simulink model "invDyn"  (R2021a)
settings: Solver=VariableStepAuto  StartTime=0.0  StopTime=60  RelTol=1e-3
values from neighbouring files (symbols this model uses):
  kd = eye(3)*40    [params.m]
  kp = eye(3)*1000    [params.m]
settings Model: Creator=antoninoparisi  LastModifiedBy=antoninoparisi
settings DebuggingCC: UnderSpecifiedDimensionMsg=warning

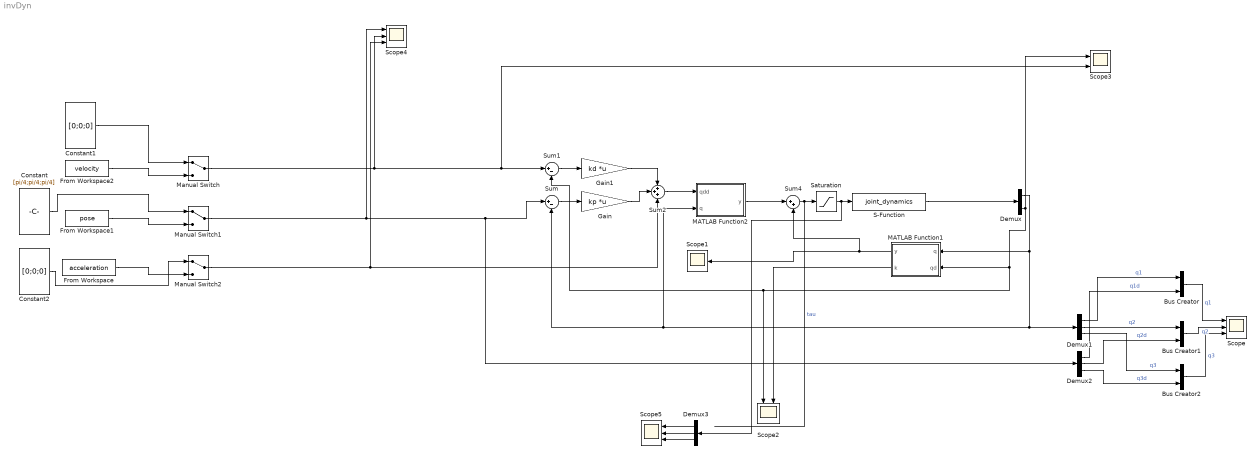
== system invDyn ==
  Bus Creator : BusCreator  Inputs=2
  Bus Creator1 : BusCreator  Inputs=2
  Bus Creator2 : BusCreator  Inputs=2
  Constant : Constant  Value=[pi/4;pi/4;pi/4]  VectorParams1D=off
  Constant1 : Constant  Value=[0;0;0]  VectorParams1D=off
  Constant2 : Constant  Value=[0;0;0]  VectorParams1D=off
  Demux : Demux  Outputs=2
  Demux1 : Demux  Outputs=3
  Demux2 : Demux  Outputs=3
  Demux3 : Demux  Outputs=3
  From Workspace : FromWorkspace  VariableName=acceleration
  From Workspace1 : FromWorkspace  VariableName=pose
  From Workspace2 : FromWorkspace  VariableName=velocity
  Gain : Gain  Gain=kp  Multiplication=Matrix(K*u) (u vector)
  Gain1 : Gain  Gain=kd  Multiplication=Matrix(K*u) (u vector)
  MATLAB Function1 : MATLAB Function  TreatAsAtomicUnit=on
  MATLAB Function2 : MATLAB Function  TreatAsAtomicUnit=on
  Manual Switch : ManualSwitch
  Manual Switch1 : ManualSwitch
  Manual Switch2 : ManualSwitch
  S-Function : S-Function  FunctionName=joint_dynamics  Parameters=robot  SFunctionDeploymentMode=off  EnableBusSupport=off
  Saturation : Saturate  UpperLimit=20  LowerLimit=-20
  Scope : Scope  NumInputPorts=3
  Scope1 : Scope
  Scope2 : Scope  NumInputPorts=2
  Scope3 : Scope  NumInputPorts=2
  Scope4 : Scope  NumInputPorts=3
  Scope5 : Scope  NumInputPorts=3
  Sum : Sum  Inputs=|+-
  Sum1 : Sum  Inputs=|+-
  Sum2 : Sum  Inputs=+++
  Sum4 : Sum  Inputs=|++
  wires:
  Demux/1 -> MATLAB Function1/1(q), Demux1/1, MATLAB Function2/2(q), Sum/2
  Manual Switch1/1 -> Scope4/1, Sum/1, Demux2/1
  Bus Creator2/1 -> Scope/3  "q3"
  Sum/1 -> Gain/1
  S-Function/1 -> Demux/1
  Demux2/1 -> Bus Creator/2  "q1d"
  Bus Creator/1 -> Scope/1  "q1"
  Bus Creator1/1 -> Scope/2  "q2"
  Demux2/3 -> Bus Creator2/2  "q3d"
  Demux1/3 -> Bus Creator2/1  "q3"
  Demux1/1 -> Bus Creator/1  "q1"
  Demux1/2 -> Bus Creator1/1  "q2"
  Demux2/2 -> Bus Creator1/2  "q2d"
  Sum1/1 -> Gain1/1
  Gain1/1 -> Sum2/1
  Gain/1 -> Sum2/2
  Sum2/1 -> MATLAB Function2/1(qdd)
  Demux/2 -> Scope3/1, MATLAB Function1/2(qd), Sum1/2, Scope2/1
  Manual Switch2/1 -> Sum2/3, Scope4/3
  MATLAB Function1/2(k) -> Scope2/2
  MATLAB Function1/1(y) -> Sum4/2, Scope1/1
  Manual Switch/1 -> Scope4/2, Scope3/2, Sum1/1
  From Workspace/1 -> Manual Switch2/2
  From Workspace1/1 -> Manual Switch1/2
  From Workspace2/1 -> Manual Switch/2
  Constant/1 -> Manual Switch1/1
  Constant1/1 -> Manual Switch/1
  Constant2/1 -> Manual Switch2/1
  MATLAB Function2/1(y) -> Sum4/1
  Demux3/1 -> Scope5/1
  Demux3/2 -> Scope5/2
  Demux3/3 -> Scope5/3
  Sum4/1 -> Saturation/1  "tau"
  Saturation/1 -> Demux3/1, S-Function/1

== matlab function invDyn/MATLAB Function2 ==
  data: qdd input size=3; y output size=3; q input size=3
function y = B_id(qdd,q)
%  y = B_Lagrangian(q)*qdd;
 y = B_hat_lagrangian(q)*qdd;

== matlab function invDyn/MATLAB Function1 ==
  data: q input size=3; y output size=3; qd input size=3; k output size=3
function [y,k] = N_id(q,qd)

% y = C_Lagrangian(q,qd)*qd+G_Lagrangian(q);
y = C_hat_lagrangian(q,qd)*qd+G_Lagrangian(q);

k = C_Lagrangian(q,qd)*qd;
